simulink model "test_utility"  (R2017a)
settings: Solver=FixedStepAuto  StartTime=0.0  StopTime=10.0  RelTol=1e-3
libraries: simulink x1
settings Model: Creator=Santy  LastModifiedBy=Santy

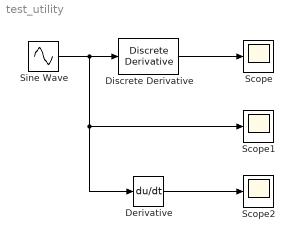
== system test_utility ==
  Derivative : Derivative  CoefficientInTFapproximation=1
  Discrete Derivative : simulink/Discrete/Discrete Derivative  gainval=1.0  ICPrevScaledInput=1  InputProcessing=Columns as channels (frame based)  OutMin=[]  OutMax=[]  OutDataType=fixdt(1, 16)  OutScaling=2^-10  DoSatur=off
  Scope : Scope
  Scope1 : Scope
  Scope2 : Scope
  Sine Wave : Sin  SampleTime=0
  wires:
  Sine Wave/1 -> Scope1/1, Derivative/1, Discrete Derivative/1
  Discrete Derivative/1 -> Scope/1
  Derivative/1 -> Scope2/1
